simulink model "Test_Byte_Demultiplexer_1_to_16"  (Simulink 8.7)
settings: Solver=ode45  StartTime=0.0  StopTime=len  RelTol=1e-3
libraries: Miscellaneous x17, Byte_Demultiplexers_Lib x1, commutil2 x1
settings Model: Creator=N  LastModifiedBy=Jozko Mrkvicka
settings DataIOCC: LimitDataPoints=off
settings DebuggingCC: UnderspecifiedInitializationDetection=Simplified  MergeDetectMultiDrivingBlocksExec=error
settings HardwareCC: ProdBitPerPointer=64  ProdLargestAtomicFloat=Float  ProdIntDivRoundTo=Zero  ProdEndianess=LittleEndian  ProdHWDeviceType=Intel->x86-64 (Windows64)
settings ModelReferenceCC: PropagateSignalLabelsOutOfModel=on

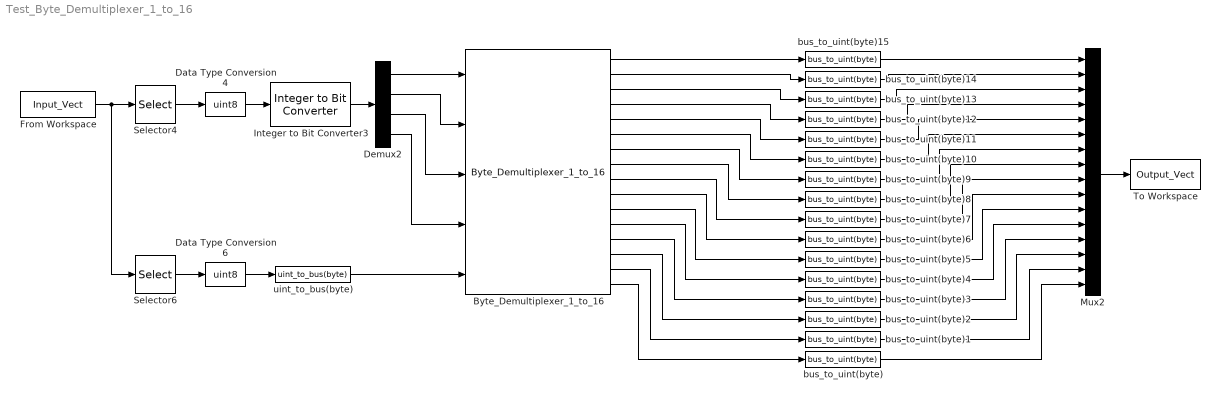
== system Test_Byte_Demultiplexer_1_to_16 ==
  Byte_Demultiplexer_1_to_16 : Byte_Demultiplexers_Lib/Byte_Demultiplexers_Lib/Byte_Demultiplexer_1_to_16
  Data Type Conversion4 : DataTypeConversion  OutDataTypeStr=uint8
  Data Type Conversion6 : DataTypeConversion  OutDataTypeStr=uint8
  Demux2 : Demux
  From Workspace : FromWorkspace  VariableName=Input_Vect  SampleTime=1  Interpolate=off  OutputAfterFinalValue=Holding final value
  Integer to Bit Converter3 : commutil2/Integer to Bit Converter  nbits=4  signedInputValues=Unsigned  bitOrder=MSB first  outDtype=boolean
  Mux2 : Mux  Inputs=16
  Selector4 : Selector  IndexMode=Zero-based  InputPortWidth=2  SampleTime=1  IndexOptions=Index vector (dialog)  Indices=0  OutputSizes=1
  Selector6 : Selector  IndexMode=Zero-based  InputPortWidth=2  IndexOptions=Index vector (dialog)  Indices=1  OutputSizes=1
  To Workspace : ToWorkspace  VariableName=Output_Vect  SampleTime=1
  bus_to_uint(byte){,1..15} (16 alike) : Miscellaneous/bus_to_uint(byte)
  uint_to_bus(byte) : Miscellaneous/uint_to_bus(byte)
  wires:
  Integer to Bit Converter3/1 -> Demux2/1
  Selector4/1 -> Data Type Conversion4/1
  Data Type Conversion4/1 -> Integer to Bit Converter3/1
  From Workspace/1 -> Selector4/1, Selector6/1
  Demux2/1 -> Byte_Demultiplexer_1_to_16/1
  Demux2/2 -> Byte_Demultiplexer_1_to_16/2
  Demux2/3 -> Byte_Demultiplexer_1_to_16/3
  Selector6/1 -> Data Type Conversion6/1
  Data Type Conversion6/1 -> uint_to_bus(byte)/1
  Mux2/1 -> To Workspace/1
  Demux2/4 -> Byte_Demultiplexer_1_to_16/4
  Byte_Demultiplexer_1_to_16/1 -> bus_to_uint(byte)15/1
  Byte_Demultiplexer_1_to_16/2 -> bus_to_uint(byte)14/1
  Byte_Demultiplexer_1_to_16/3 -> bus_to_uint(byte)13/1
  Byte_Demultiplexer_1_to_16/4 -> bus_to_uint(byte)12/1
  Byte_Demultiplexer_1_to_16/5 -> bus_to_uint(byte)11/1
  Byte_Demultiplexer_1_to_16/6 -> bus_to_uint(byte)10/1
  Byte_Demultiplexer_1_to_16/7 -> bus_to_uint(byte)9/1
  Byte_Demultiplexer_1_to_16/8 -> bus_to_uint(byte)8/1
  Byte_Demultiplexer_1_to_16/9 -> bus_to_uint(byte)7/1
  Byte_Demultiplexer_1_to_16/10 -> bus_to_uint(byte)6/1
  Byte_Demultiplexer_1_to_16/11 -> bus_to_uint(byte)5/1
  Byte_Demultiplexer_1_to_16/12 -> bus_to_uint(byte)4/1
  Byte_Demultiplexer_1_to_16/13 -> bus_to_uint(byte)3/1
  Byte_Demultiplexer_1_to_16/14 -> bus_to_uint(byte)2/1
  Byte_Demultiplexer_1_to_16/15 -> bus_to_uint(byte)1/1
  Byte_Demultiplexer_1_to_16/16 -> bus_to_uint(byte)/1
  uint_to_bus(byte)/1 -> Byte_Demultiplexer_1_to_16/5
  bus_to_uint(byte)/1 -> Mux2/16
  bus_to_uint(byte)1/1 -> Mux2/15
  bus_to_uint(byte)2/1 -> Mux2/14
  bus_to_uint(byte)3/1 -> Mux2/13
  bus_to_uint(byte)4/1 -> Mux2/12
  bus_to_uint(byte)5/1 -> Mux2/11
  bus_to_uint(byte)6/1 -> Mux2/10
  bus_to_uint(byte)7/1 -> Mux2/9
  bus_to_uint(byte)8/1 -> Mux2/8
  bus_to_uint(byte)9/1 -> Mux2/7
  bus_to_uint(byte)10/1 -> Mux2/6
  bus_to_uint(byte)11/1 -> Mux2/5
  bus_to_uint(byte)12/1 -> Mux2/4
  bus_to_uint(byte)13/1 -> Mux2/3
  bus_to_uint(byte)14/1 -> Mux2/2
  bus_to_uint(byte)15/1 -> Mux2/1
